simulink model "capsubot_Simulation_comparison_LandC"  (R2019a)
settings: Solver=ode45  StartTime=0.0  StopTime=16  FixedStep=.0001  MaxStep=.001  MinStep=.000001  RelTol=1e-3  EnableMultiTasking=on
values from neighbouring files (symbols this model uses):
  a1 = -a_stoke    [capsubot_dataperfectLuGree.m]
  a_c_desired_backward = [-a_all1' -a_all2']    [capsubot_dataperfectLuGree.m]
  a_u_desired = [a_all2' a_all1' a_all1' a_all2']    [capsubot_dataperfectLuGree.m]
  a_u_desired_backward = [-a_all2' -a_all1' -a_all1' -a_all2']    [capsubot_dataperfectLuGree.m]
  f_sm = data(8)    [capsubot_dataperfectLuGree.m]
  f_sM = 0.49    [capsubot_dataperfectLuGree.m]
  fv_Cap = data(9)    [capsubot_dataperfectLuGree.m]
  fv_IM = data(9)    [capsubot_dataperfectLuGree.m]
  g = 9.8    [capsubot_dataperfectLuGree.m]
  j = 30    [capsubot_dataperfectLuGree.m]
  k1 = 300    [capsubot_dataperfectLuGree.m]
  k2 = 100    [capsubot_dataperfectLuGree.m]
  m = data(2)    [capsubot_dataperfectLuGree.m]
  M = data(1)    [capsubot_dataperfectLuGree.m]
  m1 = data(2)    [capsubot_dataperfectLuGree.m]
  mu = data(3)    [capsubot_dataperfectLuGree.m]
  mu_1 = data(4)    [capsubot_dataperfectLuGree.m]
  mu_m = data(4)    [capsubot_dataperfectLuGree.m]
  sig_cap0 = data(8)    [capsubot_dataperfectLuGree.m]
  sig_cap1 = data(11)    [capsubot_dataperfectLuGree.m]
  sig_IM0 = data(8)    [capsubot_dataperfectLuGree.m]
  sig_IM1 = data(9)    [capsubot_dataperfectLuGree.m]
  tc = zeros(n,2)    [capsubot_dataperfectLuGree.m]
  tu = zeros(n,4)    [capsubot_dataperfectLuGree.m]
  z_cap = data(7)    [capsubot_dataperfectLuGree.m]
  z_IM = data(9)    [capsubot_dataperfectLuGree.m]
undefined symbols (not defined in the file or in its folder): profile, time_sim_individual_cum
libraries: fuzblock x2
(part 2 of 3)

== matlab function capsubot_Simulation_comparison_LandC/ Trajectory Tracking Controller/Selection Algorithm/Embedded MATLAB Function for the selection of acceleration	 ==
  data: u input; a_md output; tu parameter; time_sim_individual_cum parameter; profile parameter; a_u_desired parameter; a_c_desired_backward parameter; tc parameter; a_u_desired_backward parameter
function a_md  = fcn(u, tu, time_sim_individual_cum,profile,a_u_desired, a_c_desired_backward, tc, a_u_desired_backward )
 
t_add1=0;

%% 11111111111111111%%%%%%%%%%%%%%       %%%%    %%%%

if u<=(t_add1 + tu(profile(1),1))
        a_md =a_u_desired(profile(1),1) ;
elseif (u>(t_add1 + tu(profile(1),1))) && (u<=(t_add1 + tu(profile(1),2))) 
        a_md =a_u_desired(profile(1),2) ;
elseif (u>(t_add1 + tu(profile(1),2))) && (u<=(t_add1 + tu(profile(1),3))) 
        a_md =a_u_desired(profile(1),3) ;
elseif (u>(t_add1 + tu(profile(1),3))) && (u<=(t_add1 + tu(profile(1),4)))
             a_md =a_u_desired(profile(1),4) ;

elseif (u>(t_add1 + tu(profile(1),4))) && (u<=(tu(profile(1),4) + tu(profile(1),1)))
             a_md =a_u_desired(profile(1),1) ;                  
elseif (u>(tu(profile(1),4) + tu(profile(1),1))) && (u<=(tu(profile(1),4) + tu(profile(1),2)))
             a_md =a_u_desired(profile(1),2) ;
elseif (u>(tu(profile(1),4) + tu(profile(1),2))) && (u<=(tu(profile(1),4) + tu(profile(1),3)))
             a_md =a_u_desired(profile(1),3) ;   
elseif (u>(tu(profile(1),4) + tu(profile(1),3))) && (u<=(tu(profile(1),4) + tu(profile(1),4)))
             a_md =a_u_desired(profile(1),4) ;      

elseif (u>( tu(profile(1),4) + tu(profile(1),4))) && (u<=(2*tu(profile(1),4) + tu(profile(1),1)))
             a_md =a_u_desired(profile(1),1) ;                  
elseif (u>(2*tu(profile(1),4) + tu(profile(1),1))) && (u<=(2*tu(profile(1),4) + tu(profile(1),2)))
             a_md =a_u_desired(profile(1),2) ;
elseif (u>(2*tu(profile(1),4) + tu(profile(1),2))) && (u<=(2*tu(profile(1),4) + tu(profile(1),3)))
             a_md =a_u_desired(profile(1),3) ;   
elseif (u>(2*tu(profile(1),4) + tu(profile(1),3))) && (u<=(2*tu(profile(1),4) + tu(profile(1),4)))
             a_md =a_u_desired(profile(1),4) ;   

elseif (u>( 3*tu(profile(1),4) )) && (u<=(3*tu(profile(1),4) + tu(profile(1),1)))
             a_md =a_u_desired(profile(1),1) ;                  
elseif (u>(3*tu(profile(1),4) + tu(profile(1),1))) && (u<=(3*tu(profile(1),4) + tu(profile(1),2)))
             a_md =a_u_desired(profile(1),2) ;
elseif (u>(3*tu(profile(1),4) + tu(profile(1),2))) && (u<=(3*tu(profile(1),4) + tu(profile(1),3)))
             a_md =a_u_desired(profile(1),3) ;   
elseif (u>(3*tu(profile(1),4) + tu(profile(1),3))) && (u<=(3*tu(profile(1),4) + tu(profile(1),4)))
             a_md =a_u_desired(profile(1),4) ;                       

elseif (u>( 4*tu(profile(1),4) )) && (u<=(4*tu(profile(1),4) + tu(profile(1),1)))
             a_md =a_u_desired(profile(1),1) ;                  
elseif (u>(4*tu(profile(1),4) + tu(profile(1),1))) && (u<=(4*tu(profile(1),4) + tu(profile(1),2)))
             a_md =a_u_desired(profile(1),2) ;
elseif (u>(4*tu(profile(1),4) + tu(profile(1),2))) && (u<=(4*tu(profile(1),4) + tu(profile(1),3)))
             a_md =a_u_desired(profile(1),3) ;   
elseif (u>(4*tu(profile(1),4) + tu(profile(1),3))) && (u<=(4*tu(profile(1),4) + tu(profile(1),4)))
             a_md =a_u_desired(profile(1),4) ;    

elseif (u>( 5*tu(profile(1),4) )) && (u<=(4*tu(profile(1),4) + tu(profile(1),1)))
             a_md =a_u_desired(profile(1),1) ;                  
elseif (u>(4*tu(profile(1),4) + tu(profile(1),1))) && (u<=(4*tu(profile(1),4) + tu(profile(1),2)))
             a_md =a_u_desired(profile(1),2) ;
elseif (u>(4*tu(profile(1),4) + tu(profile(1),2))) && (u<=(4*tu(profile(1),4) + tu(profile(1),3)))
             a_md =a_u_desired(profile(1),3) ;   
elseif (u>(4*tu(profile(1),4) + tu(profile(1),3))) && (u<=(4*tu(profile(1),4) + tu(profile(1),4)))
             a_md =a_u_desired(profile(1),4) ;   


             
%% 22222222222222222 %%%%%%%%%%%%%%       %%%%    %%%%



elseif (u>( time_sim_individual_cum (1) )) && (u<=( time_sim_individual_cum(1) + tu(profile(2),1)))
             a_md =a_u_desired(profile(2),1) ;                  
elseif (u>( time_sim_individual_cum (1) + tu(profile(2),1) )) && (u<=( time_sim_individual_cum(1) + tu(profile(2),2)))
             a_md =a_u_desired(profile(2),2) ;
elseif (u>( time_sim_individual_cum (1) + tu(profile(2),2) )) && (u<=( time_sim_individual_cum(1) + tu(profile(2),3)))
             a_md =a_u_desired(profile(2),3) ;   
elseif (u>( time_sim_individual_cum (1) + tu(profile(2),3) )) && (u<=( time_sim_individual_cum(1) + tu(profile(2),4)))
             a_md =a_u_desired(profile(2),4) ;  

elseif (u>( time_sim_individual_cum (1) + 1*tu(profile(2),4) )) && (u<=(time_sim_individual_cum(1) + 1*tu(profile(2),4) + tu(profile(2),1)))
             a_md =a_u_desired(profile(2),1) ;                  
elseif (u>( time_sim_individual_cum (1) + 1*tu(profile(2),4) + tu(profile(2),1) )) && (u<=( time_sim_individual_cum(1) + 1*tu(profile(2),4) + tu(profile(2),2)))
             a_md =a_u_desired(profile(2),2) ;
elseif (u>( time_sim_individual_cum (1)+ 1*tu(profile(2),4) + tu(profile(2),2) )) && (u<=( time_sim_individual_cum(1)+ 1*tu(profile(2),4) + tu(profile(2),3)))
             a_md =a_u_desired(profile(2),3) ;   
elseif (u>( time_sim_individual_cum (1)+ 1*tu(profile(2),4) + tu(profile(2),3) )) && (u<=( time_sim_individual_cum(1)+ 1*tu(profile(2),4) + tu(profile(2),4)))
             a_md =a_u_desired(profile(2),4) ;                       


elseif (u>( time_sim_individual_cum (1) + 2*tu(profile(2),4) )) && (u<=(time_sim_individual_cum(1) + 2*tu(profile(2),4) + tu(profile(2),1)))
             a_md =a_u_desired(profile(2),1) ;                  
elseif (u>( time_sim_individual_cum (1) + 2*tu(profile(2),4) + tu(profile(2),1) )) && (u<=( time_sim_individual_cum(1) + 2*tu(profile(2),4) + tu(profile(2),2)))
             a_md =a_u_desired(profile(2),2) ;
elseif (u>( time_sim_individual_cum (1)+ 2*tu(profile(2),4) + tu(profile(2),2) )) && (u<=( time_sim_individual_cum(1)+ 2*tu(profile(2),4) + tu(profile(2),3)))
             a_md =a_u_desired(profile(2),3) ;   
elseif (u>( time_sim_individual_cum (1)+ 2*tu(profile(2),4) + tu(profile(2),3) )) && (u<=( time_sim_individual_cum(1)+ 2*tu(profile(2),4) + tu(profile(2),4)))
             a_md =a_u_desired(profile(2),4) ;                       
             

elseif (u>( time_sim_individual_cum (1) + 3*tu(profile(2),4) )) && (u<=(time_sim_individual_cum(1) + 3*tu(profile(2),4) + tu(profile(2),1)))
             a_md =a_u_desired(profile(2),1) ;                  
elseif (u>( time_sim_individual_cum (1) + 3*tu(profile(2),4) + tu(profile(2),1) )) && (u<=( time_sim_individual_cum(1) + 3*tu(profile(2),4) + tu(profile(2),2)))
             a_md =a_u_desired(profile(2),2) ;
elseif (u>( time_sim_individual_cum (1)+ 3*tu(profile(2),4) + tu(profile(2),2) )) && (u<=( time_sim_individual_cum(1)+ 3*tu(profile(2),4) + tu(profile(2),3)))
             a_md =a_u_desired(profile(2),3) ;   
elseif (u>( time_sim_individual_cum (1)+ 3*tu(profile(2),4) + tu(profile(2),3) )) && (u<=( time_sim_individual_cum(1)+ 3*tu(profile(2),4) + tu(profile(2),4)))
             a_md =a_u_desired(profile(2),4) ;               
             
             
elseif (u>( time_sim_individual_cum (1) + 4*tu(profile(2),4) )) && (u<=(time_sim_individual_cum(1) + 4*tu(profile(2),4) + tu(profile(2),1)))
             a_md =a_u_desired(profile(2),1) ;                  
elseif (u>( time_sim_individual_cum (1) + 4*tu(profile(2),4) + tu(profile(2),1) )) && (u<=( time_sim_individual_cum(1) + 4*tu(profile(2),4) + tu(profile(2),2)))
             a_md =a_u_desired(profile(2),2) ;
elseif (u>( time_sim_individual_cum (1)+ 4*tu(profile(2),4) + tu(profile(2),2) )) && (u<=( time_sim_individual_cum(1)+ 4*tu(profile(2),4) + tu(profile(2),3)))
             a_md =a_u_desired(profile(2),3) ;   
elseif (u>( time_sim_individual_cum (1)+ 4*tu(profile(2),4) + tu(profile(2),3) )) && (u<=( time_sim_individual_cum(1)+ 4*tu(profile(2),4) + tu(profile(2),4)))
             a_md =a_u_desired(profile(2),4) ; 
             
             

%% 33333333333333333333 %%%%%%%%%%%%%%       %%%%    %%%%             

             

elseif (u>( time_sim_individual_cum (2) + 0*tu(profile(3),4) )) && (u<=(time_sim_individual_cum(2) + 0*tu(profile(3),4) + tu(profile(3),1)))
             a_md =a_u_desired(profile(3),1) ;                  
elseif (u>( time_sim_individual_cum (2) + 0*tu(profile(3),4) + tu(profile(3),1) )) && (u<=( time_sim_individual_cum(2) + 0*tu(profile(3),4) + tu(profile(3),2)))
             a_md =a_u_desired(profile(3),2) ;
elseif (u>( time_sim_individual_cum (2)+ 0*tu(profile(3),4) + tu(profile(3),2) )) && (u<=( time_sim_individual_cum(2)+ 0*tu(profile(3),4) + tu(profile(3),3)))
             a_md =a_u_desired(profile(3),3) ;   
elseif (u>( time_sim_individual_cum (2)+ 0*tu(profile(3),4) + tu(profile(3),3) )) && (u<=( time_sim_individual_cum(2)+ 0*tu(profile(3),4) + tu(profile(3),4)))
             a_md =a_u_desired(profile(3),4) ;    
             
             
elseif (u>( time_sim_individual_cum (2) + 1*tu(profile(3),4) )) && (u<=(time_sim_individual_cum(2) + 1*tu(profile(3),4) + tu(profile(3),1)))
             a_md =a_u_desired(profile(3),1) ;                  
elseif (u>( time_sim_individual_cum (2) + 1*tu(profile(3),4) + tu(profile(3),1) )) && (u<=( time_sim_individual_cum(2) + 1*tu(profile(3),4) + tu(profile(3),2)))
             a_md =a_u_desired(profile(3),2) ;
elseif (u>( time_sim_individual_cum (2)+ 1*tu(profile(3),4) + tu(profile(3),2) )) && (u<=( time_sim_individual_cum(2)+ 1*tu(profile(3),4) + tu(profile(3),3)))
             a_md =a_u_desired(profile(3),3) ;   
elseif (u>( time_sim_individual_cum (2)+ 1*tu(profile(3),4) + tu(profile(3),3) )) && (u<=( time_sim_individual_cum(2)+ 1*tu(profile(3),4) + tu(profile(3),4)))
             a_md =a_u_desired(profile(3),4) ;     
             
             
elseif (u>( time_sim_individual_cum (2) + 2*tu(profile(3),4) )) && (u<=(time_sim_individual_cum(2) + 2*tu(profile(3),4) + tu(profile(3),1)))
             a_md =a_u_desired(profile(3),1) ;                  
elseif (u>( time_sim_individual_cum (2) + 2*tu(profile(3),4) + tu(profile(3),1) )) && (u<=( time_sim_individual_cum(2) + 2*tu(profile(3),4) + tu(profile(3),2)))
             a_md =a_u_desired(profile(3),2) ;
elseif (u>( time_sim_individual_cum (2)+ 2*tu(profile(3),4) + tu(profile(3),2) )) && (u<=( time_sim_individual_cum(2)+ 2*tu(profile(3),4) + tu(profile(3),3)))
             a_md =a_u_desired(profile(3),3) ;   
elseif (u>( time_sim_individual_cum (2)+ 2*tu(profile(3),4) + tu(profile(3),3) )) && (u<=( time_sim_individual_cum(2)+ 2*tu(profile(3),4) + tu(profile(3),4)))
             a_md =a_u_desired(profile(3),4) ;                
             
             
elseif (u>( time_sim_individual_cum (2) + 3*tu(profile(3),4) )) && (u<=(time_sim_individual_cum(2) + 3*tu(profile(3),4) + tu(profile(3),1)))
             a_md =a_u_desired(profile(3),1) ;                  
elseif (u>( time_sim_individual_cum (2) + 3*tu(profile(3),4) + tu(profile(3),1) )) && (u<=( time_sim_individual_cum(2) + 3*tu(profile(3),4) + tu(profile(3),2)))
             a_md =a_u_desired(profile(3),2) ;
elseif (u>( time_sim_individual_cum (2)+ 3*tu(profile(3),4) + tu(profile(3),2) )) && (u<=( time_sim_individual_cum(2)+ 3*tu(profile(3),4) + tu(profile(3),3)))
             a_md =a_u_desired(profile(3),3) ;   
elseif (u>( time_sim_individual_cum (2)+ 3*tu(profile(3),4) + tu(profile(3),3) )) && (u<=( time_sim_individual_cum(2)+ 3*tu(profile(3),4) + tu(profile(3),4)))
             a_md =a_u_desired(profile(3),4) ;   
             
             
elseif (u>( time_sim_individual_cum (2) + 4*tu(profile(3),4) )) && (u<=(time_sim_individual_cum(2) + 4*tu(profile(3),4) + tu(profile(3),1)))
             a_md =a_u_desired(profile(3),1) ;                  
elseif (u>( time_sim_individual_cum (2) + 4*tu(profile(3),4) + tu(profile(3),1) )) && (u<=( time_sim_individual_cum(2) + 4*tu(profile(3),4) + tu(profile(3),2)))
             a_md =a_u_desired(profile(3),2) ;
elseif (u>( time_sim_individual_cum (2)+ 4*tu(profile(3),4) + tu(profile(3),2) )) && (u<=( time_sim_individual_cum(2)+ 4*tu(profile(3),4) + tu(profile(3),3)))
             a_md =a_u_desired(profile(3),3) ;   
elseif (u>( time_sim_individual_cum (2)+ 4*tu(profile(3),4) + tu(profile(3),3) )) && (u<=( time_sim_individual_cum(2)+ 4*tu(profile(3),4) + tu(profile(3),4)))
             a_md =a_u_desired(profile(3),4) ;  
             
             
             
             
%% 44444444444444444444 %%%%%%%%%%%%%%       %%%%    %%%%               
             
             
             
             
elseif (u>( time_sim_individual_cum (3) + 0*tu(profile(4),4) )) && (u<=(time_sim_individual_cum(3) + 0*tu(profile(4),4) + tu(profile(4),1)))
             a_md =a_u_desired(profile(4),1) ;                  
elseif (u>( time_sim_individual_cum (3) + 0*tu(profile(4),4) + tu(profile(4),1) )) && (u<=( time_sim_individual_cum(3) + 0*tu(profile(4),4) + tu(profile(4),2)))
             a_md =a_u_desired(profile(4),2) ;
elseif (u>( time_sim_individual_cum (3)+ 0*tu(profile(4),4) + tu(profile(4),2) )) && (u<=( time_sim_individual_cum(3)+ 0*tu(profile(4),4) + tu(profile(4),3)))
             a_md =a_u_desired(profile(4),3) ;   
elseif (u>( time_sim_individual_cum (3)+ 0*tu(profile(4),4) + tu(profile(4),3) )) && (u<=( time_sim_individual_cum(3)+ 0*tu(profile(4),4) + tu(profile(4),4)))
             a_md =a_u_desired(profile(4),4) ;               
             
             
elseif (u>( time_sim_individual_cum (3) + 1*tu(profile(4),4) )) && (u<=(time_sim_individual_cum(3) + 1*tu(profile(4),4) + tu(profile(4),1)))
             a_md =a_u_desired(profile(4),1) ;                  
elseif (u>( time_sim_individual_cum (3) + 1*tu(profile(4),4) + tu(profile(4),1) )) && (u<=( time_sim_individual_cum(3) + 1*tu(profile(4),4) + tu(profile(4),2)))
             a_md =a_u_desired(profile(4),2) ;
elseif (u>( time_sim_individual_cum (3)+ 1*tu(profile(4),4) + tu(profile(4),2) )) && (u<=( time_sim_individual_cum(3)+ 1*tu(profile(4),4) + tu(profile(4),3)))
             a_md =a_u_desired(profile(4),3) ;   
elseif (u>( time_sim_individual_cum (3)+ 1*tu(profile(4),4) + tu(profile(4),3) )) && (u<=( time_sim_individual_cum(3)+ 1*tu(profile(4),4) + tu(profile(4),4)))
             a_md =a_u_desired(profile(4),4) ;   
             

elseif (u>( time_sim_individual_cum (3) + 2*tu(profile(4),4) )) && (u<=(time_sim_individual_cum(3) + 2*tu(profile(4),4) + tu(profile(4),1)))
             a_md =a_u_desired(profile(4),1) ;                  
elseif (u>( time_sim_individual_cum (3) + 2*tu(profile(4),4) + tu(profile(4),1) )) && (u<=( time_sim_individual_cum(3) + 2*tu(profile(4),4) + tu(profile(4),2)))
             a_md =a_u_desired(profile(4),2) ;
elseif (u>( time_sim_individual_cum (3)+ 2*tu(profile(4),4) + tu(profile(4),2) )) && (u<=( time_sim_individual_cum(3)+ 2*tu(profile(4),4) + tu(profile(4),3)))
             a_md =a_u_desired(profile(4),3) ;   
elseif (u>( time_sim_individual_cum (3)+ 2*tu(profile(4),4) + tu(profile(4),3) )) && (u<=( time_sim_individual_cum(3)+ 2*tu(profile(4),4) + tu(profile(4),4)))
             a_md =a_u_desired(profile(4),4) ;                
    
             
elseif (u>( time_sim_individual_cum (3) + 3*tu(profile(4),4) )) && (u<=(time_sim_individual_cum(3) + 3*tu(profile(4),4) + tu(profile(4),1)))
             a_md =a_u_desired(profile(4),1) ;                  
elseif (u>( time_sim_individual_cum (3) + 3*tu(profile(4),4) + tu(profile(4),1) )) && (u<=( time_sim_individual_cum(3) + 3*tu(profile(4),4) + tu(profile(4),2)))
             a_md =a_u_desired(profile(4),2) ;
elseif (u>( time_sim_individual_cum (3)+ 3*tu(profile(4),4) + tu(profile(4),2) )) && (u<=( time_sim_individual_cum(3)+ 3*tu(profile(4),4) + tu(profile(4),3)))
             a_md =a_u_desired(profile(4),3) ;   
elseif (u>( time_sim_individual_cum (3)+ 3*tu(profile(4),4) + tu(profile(4),3) )) && (u<=( time_sim_individual_cum(3)+ 3*tu(profile(4),4) + tu(profile(4),4)))
             a_md =a_u_desired(profile(4),4) ;                
             
             
             
%% 5555555555555555555555 %%%%%%%%%%%%%%       %%%%    %%%%               
             
             

elseif (u>( time_sim_individual_cum (4) + 0*tu(profile(5),4) )) && (u<=(time_sim_individual_cum(4) + 0*tu(profile(5),4) + tu(profile(5),1)))
             a_md =a_u_desired(profile(5),1) ;                  
elseif (u>( time_sim_individual_cum (4) + 0*tu(profile(5),4) + tu(profile(5),1) )) && (u<=( time_sim_individual_cum(4) + 0*tu(profile(5),4) + tu(profile(5),2)))
             a_md =a_u_desired(profile(5),2) ;
elseif (u>( time_sim_individual_cum (4)+ 0*tu(profile(5),4) + tu(profile(5),2) )) && (u<=( time_sim_individual_cum(4)+ 0*tu(profile(5),4) + tu(profile(5),3)))
             a_md =a_u_desired(profile(5),3) ;   
elseif (u>( time_sim_individual_cum (4)+ 0*tu(profile(5),4) + tu(profile(5),3) )) && (u<=( time_sim_individual_cum(4)+ 0*tu(profile(5),4) + tu(profile(5),4)))
             a_md =a_u_desired(profile(5),4) ;                 
             

elseif (u>( time_sim_individual_cum (4) + 1*tu(profile(5),4) )) && (u<=(time_sim_individual_cum(4) + 1*tu(profile(5),4) + tu(profile(5),1)))
             a_md =a_u_desired(profile(5),1) ;                  
elseif (u>( time_sim_individual_cum (4) + 1*tu(profile(5),4) + tu(profile(5),1) )) && (u<=( time_sim_individual_cum(4) + 1*tu(profile(5),4) + tu(profile(5),2)))
             a_md =a_u_desired(profile(5),2) ;
elseif (u>( time_sim_individual_cum (4)+ 1*tu(profile(5),4) + tu(profile(5),2) )) && (u<=( time_sim_individual_cum(4)+ 1*tu(profile(5),4) + tu(profile(5),3)))
             a_md =a_u_desired(profile(5),3) ;   
elseif (u>( time_sim_individual_cum (4)+ 1*tu(profile(5),4) + tu(profile(5),3) )) && (u<=( time_sim_individual_cum(4)+ 1*tu(profile(5),4) + tu(profile(5),4)))
             a_md =a_u_desired(profile(5),4) ;    

             
elseif (u>( time_sim_individual_cum (4) + 2*tu(profile(5),4) )) && (u<=(time_sim_individual_cum(4) + 2*tu(profile(5),4) + tu(profile(5),1)))
             a_md =a_u_desired(profile(5),1) ;                  
elseif (u>( time_sim_individual_cum (4) + 2*tu(profile(5),4) + tu(profile(5),1) )) && (u<=( time_sim_individual_cum(4) + 2*tu(profile(5),4) + tu(profile(5),2)))
             a_md =a_u_desired(profile(5),2) ;
elseif (u>( time_sim_individual_cum (4)+ 2*tu(profile(5),4) + tu(profile(5),2) )) && (u<=( time_sim_individual_cum(4)+ 2*tu(profile(5),4) + tu(profile(5),3)))
             a_md =a_u_desired(profile(5),3) ;   
elseif (u>( time_sim_individual_cum (4)+ 2*tu(profile(5),4) + tu(profile(5),3) )) && (u<=( time_sim_individual_cum(4)+ 2*tu(profile(5),4) + tu(profile(5),4)))
             a_md =a_u_desired(profile(5),4) ;              

             
elseif (u>( time_sim_individual_cum (4) + 3*tu(profile(5),4) )) && (u<=(time_sim_individual_cum(4) + 3*tu(profile(5),4) + tu(profile(5),1)))
             a_md =a_u_desired(profile(5),1) ;                  
elseif (u>( time_sim_individual_cum (4) + 3*tu(profile(5),4) + tu(profile(5),1) )) && (u<=( time_sim_individual_cum(4) + 3*tu(profile(5),4) + tu(profile(5),2)))
             a_md =a_u_desired(profile(5),2) ;
elseif (u>( time_sim_individual_cum (4)+ 3*tu(profile(5),4) + tu(profile(5),2) )) && (u<=( time_sim_individual_cum(4)+ 3*tu(profile(5),4) + tu(profile(5),3)))
             a_md =a_u_desired(profile(5),3) ;   
elseif (u>( time_sim_individual_cum (4)+ 3*tu(profile(5),4) + tu(profile(5),3) )) && (u<=( time_sim_individual_cum(4)+ 3*tu(profile(5),4) + tu(profile(5),4)))
             a_md =a_u_desired(profile(5),4) ;     
             

elseif (u>( time_sim_individual_cum (4) + 4*tu(profile(5),4) )) && (u<=(time_sim_individual_cum(4) + 4*tu(profile(5),4) + tu(profile(5),1)))
             a_md =a_u_desired(profile(5),1) ;                  
elseif (u>( time_sim_individual_cum (4) + 4*tu(profile(5),4) + tu(profile(5),1) )) && (u<=( time_sim_individual_cum(4) + 4*tu(profile(5),4) + tu(profile(5),2)))
             a_md =a_u_desired(profile(5),2) ;
elseif (u>( time_sim_individual_cum (4)+ 4*tu(profile(5),4) + tu(profile(5),2) )) && (u<=( time_sim_individual_cum(4)+ 4*tu(profile(5),4) + tu(profile(5),3)))
             a_md =a_u_desired(profile(5),3) ;   
elseif (u>( time_sim_individual_cum (4)+ 4*tu(profile(5),4) + tu(profile(5),3) )) && (u<=( time_sim_individual_cum(4)+ 4*tu(profile(5),4) + tu(profile(5),4)))
             a_md =a_u_desired(profile(5),4) ;    
             

             
%% 66666666666666666666 %%%%%%%%%%%%%%       %%%%    %%%%              
             
             
elseif (u>( time_sim_individual_cum (5) + 0*tu(profile(6),4) )) && (u<=(time_sim_individual_cum(5) + 0*tu(profile(6),4) + tu(profile(6),1)))
             a_md =a_u_desired(profile(6),1) ;                  
elseif (u>( time_sim_individual_cum (5) + 0*tu(profile(6),4) + tu(profile(6),1) )) && (u<=( time_sim_individual_cum(5) + 0*tu(profile(6),4) + tu(profile(6),2)))
             a_md =a_u_desired(profile(6),2) ;
elseif (u>( time_sim_individual_cum (5)+ 0*tu(profile(6),4) + tu(profile(6),2) )) && (u<=( time_sim_individual_cum(5)+ 0*tu(profile(6),4) + tu(profile(6),3)))
             a_md =a_u_desired(profile(6),3) ;   
elseif (u>( time_sim_individual_cum (5)+ 0*tu(profile(6),4) + tu(profile(6),3) )) && (u<=( time_sim_individual_cum(5)+ 0*tu(profile(6),4) + tu(profile(6),4)))
             a_md =a_u_desired(profile(6),4) ;   
             

elseif (u>( time_sim_individual_cum (5) + 1*tu(profile(6),4) )) && (u<=(time_sim_individual_cum(5) + 1*tu(profile(6),4) + tu(profile(6),1)))
             a_md =a_u_desired(profile(6),1) ;                  
elseif (u>( time_sim_individual_cum (5) + 1*tu(profile(6),4) + tu(profile(6),1) )) && (u<=( time_sim_individual_cum(5) + 1*tu(profile(6),4) + tu(profile(6),2)))
             a_md =a_u_desired(profile(6),2) ;
elseif (u>( time_sim_individual_cum (5)+ 1*tu(profile(6),4) + tu(profile(6),2) )) && (u<=( time_sim_individual_cum(5)+ 1*tu(profile(6),4) + tu(profile(6),3)))
             a_md =a_u_desired(profile(6),3) ;   
elseif (u>( time_sim_individual_cum (5)+ 1*tu(profile(6),4) + tu(profile(6),3) )) && (u<=( time_sim_individual_cum(5)+ 1*tu(profile(6),4) + tu(profile(6),4)))
             a_md =a_u_desired(profile(6),4) ;    
             
             
elseif (u>( time_sim_individual_cum (5) + 2*tu(profile(6),4) )) && (u<=(time_sim_individual_cum(5) + 2*tu(profile(6),4) + tu(profile(6),1)))
             a_md =a_u_desired(profile(6),1) ;                  
elseif (u>( time_sim_individual_cum (5) + 2*tu(profile(6),4) + tu(profile(6),1) )) && (u<=( time_sim_individual_cum(5) + 2*tu(profile(6),4) + tu(profile(6),2)))
             a_md =a_u_desired(profile(6),2) ;
elseif (u>( time_sim_individual_cum (5)+ 2*tu(profile(6),4) + tu(profile(6),2) )) && (u<=( time_sim_individual_cum(5)+ 2*tu(profile(6),4) + tu(profile(6),3)))
             a_md =a_u_desired(profile(6),3) ;   
elseif (u>( time_sim_individual_cum (5)+ 2*tu(profile(6),4) + tu(profile(6),3) )) && (u<=( time_sim_individual_cum(5)+ 2*tu(profile(6),4) + tu(profile(6),4)))
             a_md =a_u_desired(profile(6),4) ; 
             
             
elseif (u>( time_sim_individual_cum (5) + 3*tu(profile(6),4) )) && (u<=(time_sim_individual_cum(5) + 3*tu(profile(6),4) + tu(profile(6),1)))
             a_md =a_u_desired(profile(6),1) ;                  
elseif (u>( time_sim_individual_cum (5) + 3*tu(profile(6),4) + tu(profile(6),1) )) && (u<=( time_sim_individual_cum(5) + 3*tu(profile(6),4) + tu(profile(6),2)))
             a_md =a_u_desired(profile(6),2) ;
elseif (u>( time_sim_individual_cum (5)+ 3*tu(profile(6),4) + tu(profile(6),2) )) && (u<=( time_sim_individual_cum(5)+ 3*tu(profile(6),4) + tu(profile(6),3)))
             a_md =a_u_desired(profile(6),3) ;   
elseif (u>( time_sim_individual_cum (5)+ 3*tu(profile(6),4) + tu(profile(6),3) )) && (u<=( time_sim_individual_cum(5)+ 3*tu(profile(6),4) + tu(profile(6),4)))
             a_md =a_u_desired(profile(6),4) ;  
             
             
elseif (u>( time_sim_individual_cum (5) + 4*tu(profile(6),4) )) && (u<=(time_sim_individual_cum(5) + 4*tu(profile(6),4) + tu(profile(6),1)))
             a_md =a_u_desired(profile(6),1) ;                  
elseif (u>( time_sim_individual_cum (5) + 4*tu(profile(6),4) + tu(profile(6),1) )) && (u<=( time_sim_individual_cum(5) + 4*tu(profile(6),4) + tu(profile(6),2)))
             a_md =a_u_desired(profile(6),2) ;
elseif (u>( time_sim_individual_cum (5)+ 4*tu(profile(6),4) + tu(profile(6),2) )) && (u<=( time_sim_individual_cum(5)+ 4*tu(profile(6),4) + tu(profile(6),3)))
             a_md =a_u_desired(profile(6),3) ;   
elseif (u>( time_sim_individual_cum (5)+ 4*tu(profile(6),4) + tu(profile(6),3) )) && (u<=( time_sim_individual_cum(5)+ 4*tu(profile(6),4) + tu(profile(6),4)))
             a_md =a_u_desired(profile(6),4) ;              
             
             
             
%% 777777777777777 %%%%%%%%%%%%%%       %%%%    %%%%              
             
             
elseif (u>( time_sim_individual_cum (6) + 0*tu(profile(7),4) )) && (u<=(time_sim_individual_cum(6) + 0*tu(profile(7),4) + tu(profile(7),1)))
             a_md =a_u_desired(profile(7),1) ;                  
elseif (u>( time_sim_individual_cum (6) + 0*tu(profile(7),4) + tu(profile(7),1) )) && (u<=( time_sim_individual_cum(6) + 0*tu(profile(7),4) + tu(profile(7),2)))
             a_md =a_u_desired(profile(7),2) ;
elseif (u>( time_sim_individual_cum (6)+ 0*tu(profile(7),4) + tu(profile(7),2) )) && (u<=( time_sim_individual_cum(6)+ 0*tu(profile(7),4) + tu(profile(7),3)))
             a_md =a_u_desired(profile(7),3) ;   
elseif (u>( time_sim_individual_cum (6)+ 0*tu(profile(7),4) + tu(profile(7),3) )) && (u<=( time_sim_individual_cum(6)+ 0*tu(profile(7),4) + tu(profile(7),4)))
             a_md =a_u_desired(profile(7),4) ; 

elseif (u>( time_sim_individual_cum (6) + 1*tu(profile(7),4) )) && (u<=(time_sim_individual_cum(6) + 1*tu(profile(7),4) + tu(profile(7),1)))
             a_md =a_u_desired(profile(7),1) ;                  
elseif (u>( time_sim_individual_cum (6) + 1*tu(profile(7),4) + tu(profile(7),1) )) && (u<=( time_sim_individual_cum(6) + 1*tu(profile(7),4) + tu(profile(7),2)))
             a_md =a_u_desired(profile(7),2) ;
elseif (u>( time_sim_individual_cum (6)+ 1*tu(profile(7),4) + tu(profile(7),2) )) && (u<=( time_sim_individual_cum(6)+ 1*tu(profile(7),4) + tu(profile(7),3)))
             a_md =a_u_desired(profile(7),3) ;   
elseif (u>( time_sim_individual_cum (6)+ 1*tu(profile(7),4) + tu(profile(7),3) )) && (u<=( time_sim_individual_cum(6)+ 1*tu(profile(7),4) + tu(profile(7),4)))
             a_md =a_u_desired(profile(7),4) ; 
             
elseif (u>( time_sim_individual_cum (6) + 2*tu(profile(7),4) )) && (u<=(time_sim_individual_cum(6) + 2*tu(profile(7),4) + tu(profile(7),1)))
             a_md =a_u_desired(profile(7),1) ;                  
elseif (u>( time_sim_individual_cum (6) + 2*tu(profile(7),4) + tu(profile(7),1) )) && (u<=( time_sim_individual_cum(6) + 2*tu(profile(7),4) + tu(profile(7),2)))
             a_md =a_u_desired(profile(7),2) ;
elseif (u>( time_sim_individual_cum (6)+ 2*tu(profile(7),4) + tu(profile(7),2) )) && (u<=( time_sim_individual_cum(6)+ 2*tu(profile(7),4) + tu(profile(7),3)))
             a_md =a_u_desired(profile(7),3) ;   
elseif (u>( time_sim_individual_cum (6)+ 2*tu(profile(7),4) + tu(profile(7),3) )) && (u<=( time_sim_individual_cum(6)+ 2*tu(profile(7),4) + tu(profile(7),4)))
             a_md =a_u_desired(profile(7),4) ;      

             
elseif (u>( time_sim_individual_cum (6) + 3*tu(profile(7),4) )) && (u<=(time_sim_individual_cum(6) + 3*tu(profile(7),4) + tu(profile(7),1)))
             a_md =a_u_desired(profile(7),1) ;                  
elseif (u>( time_sim_individual_cum (6) + 3*tu(profile(7),4) + tu(profile(7),1) )) && (u<=( time_sim_individual_cum(6) + 3*tu(profile(7),4) + tu(profile(7),2)))
             a_md =a_u_desired(profile(7),2) ;
elseif (u>( time_sim_individual_cum (6)+ 3*tu(profile(7),4) + tu(profile(7),2) )) && (u<=( time_sim_individual_cum(6)+ 3*tu(profile(7),4) + tu(profile(7),3)))
             a_md =a_u_desired(profile(7),3) ;   
elseif (u>( time_sim_individual_cum (6)+ 3*tu(profile(7),4) + tu(profile(7),3) )) && (u<=( time_sim_individual_cum(6)+ 3*tu(profile(7),4) + tu(profile(7),4)))
             a_md =a_u_desired(profile(7),4) ;             
             
             

%% 88888888888888888888 %%%%%%%%%%%%%%       %%%%    %%%%              
                          
elseif (u>(time_sim_individual_cum (7) + 0*tu(profile(8),4) )) && (u<=(time_sim_individual_cum(7) + 0*tu(profile(7),4) + tu(profile(8),1)))
             a_md =a_u_desired(profile(8),1) ;                  
elseif (u>( time_sim_individual_cum (7) + 0*tu(profile(8),4) + tu(profile(8),1) )) && (u<=( time_sim_individual_cum(7) + 0*tu(profile(8),4) + tu(profile(8),2)))
             a_md =a_u_desired(profile(8),2) ;
elseif (u>( time_sim_individual_cum (7)+ 0*tu(profile(8),4) + tu(profile(8),2) )) && (u<=( time_sim_individual_cum(7)+ 0*tu(profile(8),4) + tu(profile(8),3)))
             a_md =a_u_desired(profile(8),3) ;   
elseif (u>( time_sim_individual_cum (7)+ 0*tu(profile(8),4) + tu(profile(8),3) )) && (u<=( time_sim_individual_cum(7)+ 0*tu(profile(8),4) + tu(profile(8),4)))
             a_md =a_u_desired(profile(8),4) ; 
             
elseif (u>(time_sim_individual_cum (7) + 1*tu(profile(8),4) )) && (u<=(time_sim_individual_cum(7) + 1*tu(profile(7),4) + tu(profile(8),1)))
             a_md =a_u_desired(profile(8),1) ;                  
elseif (u>( time_sim_individual_cum (7) + 1*tu(profile(8),4) + tu(profile(8),1) )) && (u<=( time_sim_individual_cum(7) + 1*tu(profile(8),4) + tu(profile(8),2)))
             a_md =a_u_desired(profile(8),2) ;
elseif (u>( time_sim_individual_cum (7)+ 1*tu(profile(8),4) + tu(profile(8),2) )) && (u<=( time_sim_individual_cum(7)+ 1*tu(profile(8),4) + tu(profile(8),3)))
             a_md =a_u_desired(profile(8),3) ;   
elseif (u>( time_sim_individual_cum (7)+ 1*tu(profile(8),4) + tu(profile(8),3) )) && (u<=( time_sim_individual_cum(7)+ 1*tu(profile(8),4) + tu(profile(8),4)))
             a_md =a_u_desired(profile(8),4) ;             
                          
elseif (u>(time_sim_individual_cum (7) + 2*tu(profile(8),4) )) && (u<=(time_sim_individual_cum(7) + 2*tu(profile(7),4) + tu(profile(8),1)))
             a_md =a_u_desired(profile(8),1) ;                  
elseif (u>( time_sim_individual_cum (7) + 2*tu(profile(8),4) + tu(profile(8),1) )) && (u<=( time_sim_individual_cum(7) + 2*tu(profile(8),4) + tu(profile(8),2)))
             a_md =a_u_desired(profile(8),2) ;
elseif (u>( time_sim_individual_cum (7)+ 2*tu(profile(8),4) + tu(profile(8),2) )) && (u<=( time_sim_individual_cum(7)+ 2*tu(profile(8),4) + tu(profile(8),3)))
             a_md =a_u_desired(profile(8),3) ;   
elseif (u>( time_sim_individual_cum (7)+ 2*tu(profile(8),4) + tu(profile(8),3) )) && (u<=( time_sim_individual_cum(7)+ 2*tu(profile(8),4) + tu(profile(8),4)))
             a_md =a_u_desired(profile(8),4) ;    
             
elseif (u>(time_sim_individual_cum (7) + 3*tu(profile(8),4) )) && (u<=(time_sim_individual_cum(7) + 3*tu(profile(7),4) + tu(profile(8),1)))
             a_md =a_u_desired(profile(8),1) ;                  
elseif (u>( time_sim_individual_cum (7) + 3*tu(profile(8),4) + tu(profile(8),1) )) && (u<=( time_sim_individual_cum(7) + 3*tu(profile(8),4) + tu(profile(8),2)))
             a_md =a_u_desired(profile(8),2) ;
elseif (u>( time_sim_individual_cum (7)+ 3*tu(profile(8),4) + tu(profile(8),2) )) && (u<=( time_sim_individual_cum(7)+ 3*tu(profile(8),4) + tu(profile(8),3)))
             a_md =a_u_desired(profile(8),3) ;   
elseif (u>( time_sim_individual_cum (7)+ 3*tu(profile(8),4) + tu(profile(8),3) )) && (u<=( time_sim_individual_cum(7)+ 3*tu(profile(8),4) + tu(profile(8),4)))
             a_md =a_u_desired(profile(8),4) ;  
             
elseif (u>(time_sim_individual_cum (7) + 4*tu(profile(8),4) )) && (u<=(time_sim_individual_cum(7) + 4*tu(profile(7),4) + tu(profile(8),1)))
             a_md =a_u_desired(profile(8),1) ;                  
elseif (u>( time_sim_individual_cum (7) + 4*tu(profile(8),4) + tu(profile(8),1) )) && (u<=( time_sim_individual_cum(7) + 4*tu(profile(8),4) + tu(profile(8),2)))
             a_md =a_u_desired(profile(8),2) ;
elseif (u>( time_sim_individual_cum (7)+ 4*tu(profile(8),4) + tu(profile(8),2) )) && (u<=( time_sim_individual_cum(7)+ 4*tu(profile(8),4) + tu(profile(8),3)))
             a_md =a_u_desired(profile(8),3) ;   
elseif (u>( time_sim_individual_cum (7)+ 4*tu(profile(8),4) + tu(profile(8),3) )) && (u<=( time_sim_individual_cum(7)+ 4*tu(profile(8),4) + tu(profile(8),4)))
             a_md =a_u_desired(profile(8),4) ;    
             
             
             
%%%%%%%%%%%%%%%%%%%%%%%%%%%%%%%%%%%%%%%%%%%%%%%%%%%%%%%%%%%%%%%%%%       
             
%% 9999999999999999999  %%%%%%%%%%%%%%       %%%%    %%%%          
             
elseif (u>(time_sim_individual_cum (8) + 0*tu(profile(8),4) )) && (u<=(time_sim_individual_cum(8) + 0*tu(profile(7),4) + tc(profile(9),1)))
             a_md =a_c_desired_backward(profile(9),1) ;                  
elseif (u>( time_sim_individual_cum (8) + 0*tu(profile(8),4) + tc(profile(8),1) )) && (u<=( time_sim_individual_cum(8) + 0*tu(profile(8),4) + tc(profile(9),2)))
             a_md =a_c_desired_backward(profile(9),2) ;

             
             
%%%%%%%%%%%%%%%%%%%%%%%%%%%%%%%%%%%%%%%%%%%%%%%%%%%%%%%%%%%%%%%%%%%      



%% 10 10 10 10 10 10  %%%%%%%%%%%%%%       %%%%    %%%% 

elseif (u>(time_sim_individual_cum (9) + 0*tu(profile(10),4) )) && (u<=(time_sim_individual_cum(9) + 0*tu(profile(10),4) + tu(profile(10),1)))
             a_md =a_u_desired_backward(profile(10),1) ;                  
elseif (u>( time_sim_individual_cum (9) + 0*tu(profile(10),4) + tu(profile(10),1) )) && (u<=( time_sim_individual_cum(9) + 0*tu(profile(10),4) + tu(profile(10),2)))
             a_md =a_u_desired_backward(profile(10),2) ;
elseif (u>( time_sim_individual_cum (9)+ 0*tu(profile(10),4) + tu(profile(10),2) )) && (u<=( time_sim_individual_cum(9)+ 0*tu(profile(10),4) + tu(profile(10),3)))
             a_md =a_u_desired_backward(profile(10),3) ;   
elseif (u>( time_sim_individual_cum (9)+ 0*tu(profile(10),4) + tu(profile(10),3) )) && (u<=( time_sim_individual_cum(9)+ 0*tu(profile(10),4) + tu(profile(10),4)))
             a_md =a_u_desired_backward(profile(10),4) ; 

elseif (u>(time_sim_individual_cum (9) + 1*tu(profile(10),4) )) && (u<=(time_sim_individual_cum(9) + 1*tu(profile(10),4) + tu(profile(10),1)))
             a_md =a_u_desired_backward(profile(10),1) ;                  
elseif (u>( time_sim_individual_cum (9) + 1*tu(profile(10),4) + tu(profile(10),1) )) && (u<=( time_sim_individual_cum(9) + 1*tu(profile(10),4) + tu(profile(10),2)))
             a_md =a_u_desired_backward(profile(10),2) ;
elseif (u>( time_sim_individual_cum (9)+ 1*tu(profile(10),4) + tu(profile(10),2) )) && (u<=( time_sim_individual_cum(9)+ 1*tu(profile(10),4) + tu(profile(10),3)))
             a_md =a_u_desired_backward(profile(10),3) ;   
elseif (u>( time_sim_individual_cum (9)+ 1*tu(profile(10),4) + tu(profile(10),3) )) && (u<=( time_sim_individual_cum(9)+ 1*tu(profile(10),4) + tu(profile(10),4)))
             a_md =a_u_desired_backward(profile(10),4) ; 
             
elseif (u>(time_sim_individual_cum (9) + 2*tu(profile(10),4) )) && (u<=(time_sim_individual_cum(9) + 2*tu(profile(10),4) + tu(profile(10),1)))
             a_md =a_u_desired_backward(profile(10),1) ;                  
elseif (u>( time_sim_individual_cum (9) + 2*tu(profile(10),4) + tu(profile(10),1) )) && (u<=( time_sim_individual_cum(9) + 2*tu(profile(10),4) + tu(profile(10),2)))
             a_md =a_u_desired_backward(profile(10),2) ;
elseif (u>( time_sim_individual_cum (9)+ 2*tu(profile(10),4) + tu(profile(10),2) )) && (u<=( time_sim_individual_cum(9)+ 2*tu(profile(10),4) + tu(profile(10),3)))
             a_md =a_u_desired_backward(profile(10),3) ;   
elseif (u>( time_sim_individual_cum (9)+ 2*tu(profile(10),4) + tu(profile(10),3) )) && (u<=( time_sim_individual_cum(9)+ 2*tu(profile(10),4) + tu(profile(10),4)))
             a_md =a_u_desired_backward(profile(10),4) ; 
             
elseif (u>(time_sim_individual_cum (9) + 3*tu(profile(10),4) )) && (u<=(time_sim_individual_cum(9) + 3*tu(profile(10),4) + tu(profile(10),1)))
             a_md =a_u_desired_backward(profile(10),1) ;                  
elseif (u>( time_sim_individual_cum (9) + 3*tu(profile(10),4) + tu(profile(10),1) )) && (u<=( time_sim_individual_cum(9) + 3*tu(profile(10),4) + tu(profile(10),2)))
             a_md =a_u_desired_backward(profile(10),2) ;
elseif (u>( time_sim_individual_cum (9)+ 3*tu(profile(10),4) + tu(profile(10),2) )) && (u<=( time_sim_individual_cum(9)+ 3*tu(profile(10),4) + tu(profile(10),3)))
             a_md =a_u_desired_backward(profile(10),3) ;   
elseif (u>( time_sim_individual_cum (9)+ 3*tu(profile(10),4) + tu(profile(10),3) )) && (u<=( time_sim_individual_cum(9)+ 3*tu(profile(10),4) + tu(profile(10),4)))
             a_md =a_u_desired_backward(profile(10),4) ;      
             
elseif (u>(time_sim_individual_cum (9) + 4*tu(profile(10),4) )) && (u<=(time_sim_individual_cum(9) + 4*tu(profile(10),4) + tu(profile(10),1)))
             a_md =a_u_desired_backward(profile(10),1) ;                  
elseif (u>( time_sim_individual_cum (9) + 4*tu(profile(10),4) + tu(profile(10),1) )) && (u<=( time_sim_individual_cum(9) + 4*tu(profile(10),4) + tu(profile(10),2)))
             a_md =a_u_desired_backward(profile(10),2) ;
elseif (u>( time_sim_individual_cum (9)+ 4*tu(profile(10),4) + tu(profile(10),2) )) && (u<=( time_sim_individual_cum(9)+ 4*tu(profile(10),4) + tu(profile(10),3)))
             a_md =a_u_desired_backward(profile(10),3) ;   
elseif (u>( time_sim_individual_cum (9)+ 4*tu(profile(10),4) + tu(profile(10),3) )) && (u<=( time_sim_individual_cum(9)+ 4*tu(profile(10),4) + tu(profile(10),4)))
             a_md =a_u_desired_backward(profile(10),4) ;              
             
elseif (u>(time_sim_individual_cum (9) + 5*tu(profile(10),4) )) && (u<=(time_sim_individual_cum(9) + 5*tu(profile(10),4) + tu(profile(10),1)))
             a_md =a_u_desired_backward(profile(10),1) ;                  
elseif (u>( time_sim_individual_cum (9) + 5*tu(profile(10),4) + tu(profile(10),1) )) && (u<=( time_sim_individual_cum(9) + 5*tu(profile(10),4) + tu(profile(10),2)))
             a_md =a_u_desired_backward(profile(10),2) ;
elseif (u>( time_sim_individual_cum (9)+ 5*tu(profile(10),4) + tu(profile(10),2) )) && (u<=( time_sim_individual_cum(9)+ 5*tu(profile(10),4) + tu(profile(10),3)))
             a_md =a_u_desired_backward(profile(10),3) ;   
elseif (u>( time_sim_individual_cum (9)+ 5*tu(profile(10),4) + tu(profile(10),3) )) && (u<=( time_sim_individual_cum(9)+ 5*tu(profile(10),4) + tu(profile(10),4)))
             a_md =a_u_desired_backward(profile(10),4) ;  
             
elseif (u>(time_sim_individual_cum (9) + 6*tu(profile(10),4) )) && (u<=(time_sim_individual_cum(9) + 6*tu(profile(10),4) + tu(profile(10),1)))
             a_md =a_u_desired_backward(profile(10),1) ;                  
elseif (u>( time_sim_individual_cum (9) + 6*tu(profile(10),4) + tu(profile(10),1) )) && (u<=( time_sim_individual_cum(9) + 6*tu(profile(10),4) + tu(profile(10),2)))
             a_md =a_u_desired_backward(profile(10),2) ;
elseif (u>( time_sim_individual_cum (9)+ 6*tu(profile(10),4) + tu(profile(10),2) )) && (u<=( time_sim_individual_cum(9)+ 6*tu(profile(10),4) + tu(profile(10),3)))
             a_md =a_u_desired_backward(profile(10),3) ;   
elseif (u>( time_sim_individual_cum (9)+ 6*tu(profile(10),4) + tu(profile(10),3) )) && (u<=( time_sim_individual_cum(9)+ 6*tu(profile(10),4) + tu(profile(10),4)))
             a_md =a_u_desired_backward(profile(10),4);  
             
elseif (u>(time_sim_individual_cum (9) + 7*tu(profile(10),4) )) && (u<=(time_sim_individual_cum(9) + 7*tu(profile(10),4) + tu(profile(10),1)))
             a_md =a_u_desired_backward(profile(10),1) ;                  
elseif (u>( time_sim_individual_cum (9) + 7*tu(profile(10),4) + tu(profile(10),1) )) && (u<=( time_sim_individual_cum(9) + 7*tu(profile(10),4) + tu(profile(10),2)))
             a_md =a_u_desired_backward(profile(10),2) ;
elseif (u>( time_sim_individual_cum (9)+ 7*tu(profile(10),4) + tu(profile(10),2) )) && (u<=( time_sim_individual_cum(9)+ 7*tu(profile(10),4) + tu(profile(10),3)))
             a_md =a_u_desired_backward(profile(10),3) ;   
elseif (u>( time_sim_individual_cum (9)+ 7*tu(profile(10),4) + tu(profile(10),3) )) && (u<=( time_sim_individual_cum(9)+ 7*tu(profile(10),4) + tu(profile(10),4)))
             a_md =a_u_desired_backward(profile(10),4) ;   
             
elseif (u>(time_sim_individual_cum (9) + 8*tu(profile(10),4) )) && (u<=(time_sim_individual_cum(9) + 8*tu(profile(10),4) + tu(profile(10),1)))
             a_md =a_u_desired_backward(profile(10),1) ;                  
elseif (u>( time_sim_individual_cum (9) + 8*tu(profile(10),4) + tu(profile(10),1) )) && (u<=( time_sim_individual_cum(9) + 8*tu(profile(10),4) + tu(profile(10),2)))
             a_md =a_u_desired_backward(profile(10),2) ;
elseif (u>( time_sim_individual_cum (9)+ 8*tu(profile(10),4) + tu(profile(10),2) )) && (u<=( time_sim_individual_cum(9)+ 8*tu(profile(10),4) + tu(profile(10),3)))
             a_md =a_u_desired_backward(profile(10),3) ;   
elseif (u>( time_sim_individual_cum (9)+ 8*tu(profile(10),4) + tu(profile(10),3) )) && (u<=( time_sim_individual_cum(9)+ 8*tu(profile(10),4) + tu(profile(10),4)))
             a_md =a_u_desired_backward(profile(10),4) ;    
             
                          
             
             
%% 11 11 11 11 11 11  %%%%%%%%%%%%%%       %%%%    %%%%              

elseif (u>(time_sim_individual_cum (10) + 0*tu(profile(11),4) )) && (u<=(time_sim_individual_cum(10) + 0*tu(profile(11),4) + tu(profile(11),1)))
             a_md =a_u_desired_backward(profile(11),1) ;                  
elseif (u>( time_sim_individual_cum (10) + 0*tu(profile(11),4) + tu(profile(11),1) )) && (u<=( time_sim_individual_cum(10) + 0*tu(profile(11),4) + tu(profile(11),2)))
             a_md =a_u_desired_backward(profile(11),2) ;
elseif (u>( time_sim_individual_cum (10)+ 0*tu(profile(11),4) + tu(profile(11),2) )) && (u<=( time_sim_individual_cum(10)+ 0*tu(profile(11),4) + tu(profile(11),3)))
             a_md =a_u_desired_backward(profile(11),3) ;   
elseif (u>( time_sim_individual_cum (10)+ 0*tu(profile(11),4) + tu(profile(11),3) )) && (u<=( time_sim_individual_cum(10)+ 0*tu(profile(11),4) + tu(profile(11),4)))
             a_md =a_u_desired_backward(profile(11),4) ;              
             
elseif (u>(time_sim_individual_cum (10) + 1*tu(profile(11),4) )) && (u<=(time_sim_individual_cum(10) + 1*tu(profile(11),4) + tu(profile(11),1)))
             a_md =a_u_desired_backward(profile(11),1) ;                  
elseif (u>( time_sim_individual_cum (10) + 1*tu(profile(11),4) + tu(profile(11),1) )) && (u<=( time_sim_individual_cum(10) + 1*tu(profile(11),4) + tu(profile(11),2)))
             a_md =a_u_desired_backward(profile(11),2) ;
elseif (u>( time_sim_individual_cum (10)+ 1*tu(profile(11),4) + tu(profile(11),2) )) && (u<=( time_sim_individual_cum(10)+ 1*tu(profile(11),4) + tu(profile(11),3)))
             a_md =a_u_desired_backward(profile(11),3) ;   
elseif (u>( time_sim_individual_cum (10)+ 1*tu(profile(11),4) + tu(profile(11),3) )) && (u<=( time_sim_individual_cum(10)+ 1*tu(profile(11),4) + tu(profile(11),4)))
             a_md =a_u_desired_backward(profile(11),4) ; 
             
elseif (u>(time_sim_individual_cum (10) + 2*tu(profile(11),4) )) && (u<=(time_sim_individual_cum(10) + 2*tu(profile(11),4) + tu(profile(11),1)))
             a_md =a_u_desired_backward(profile(11),1) ;                  
elseif (u>( time_sim_individual_cum (10) + 2*tu(profile(11),4) + tu(profile(11),1) )) && (u<=( time_sim_individual_cum(10) + 2*tu(profile(11),4) + tu(profile(11),2)))
             a_md =a_u_desired_backward(profile(11),2) ;
elseif (u>( time_sim_individual_cum (10)+ 2*tu(profile(11),4) + tu(profile(11),2) )) && (u<=( time_sim_individual_cum(10)+ 2*tu(profile(11),4) + tu(profile(11),3)))
             a_md =a_u_desired_backward(profile(11),3) ;   
elseif (u>( time_sim_individual_cum (10)+ 2*tu(profile(11),4) + tu(profile(11),3) )) && (u<=( time_sim_individual_cum(10)+ 2*tu(profile(11),4) + tu(profile(11),4)))
             a_md =a_u_desired_backward(profile(11),4) ;               
             
elseif (u>(time_sim_individual_cum (10) + 3*tu(profile(11),4) )) && (u<=(time_sim_individual_cum(10) + 3*tu(profile(11),4) + tu(profile(11),1)))
             a_md =a_u_desired_backward(profile(11),1) ;                  
elseif (u>( time_sim_individual_cum (10) + 3*tu(profile(11),4) + tu(profile(11),1) )) && (u<=( time_sim_individual_cum(10) + 3*tu(profile(11),4) + tu(profile(11),2)))
             a_md =a_u_desired_backward(profile(11),2) ;
elseif (u>( time_sim_individual_cum (10)+ 3*tu(profile(11),4) + tu(profile(11),2) )) && (u<=( time_sim_individual_cum(10)+ 3*tu(profile(11),4) + tu(profile(11),3)))
             a_md =a_u_desired_backward(profile(11),3) ;   
elseif (u>( time_sim_individual_cum (10)+ 3*tu(profile(11),4) + tu(profile(11),3) )) && (u<=( time_sim_individual_cum(10)+ 3*tu(profile(11),4) + tu(profile(11),4)))
             a_md =a_u_desired_backward(profile(11),4) ; 
             
             
%% 12 12 12 12 12 12  %%%%%%%%%%%%%%       %%%%    %%%%              
             
elseif (u>(time_sim_individual_cum (11) + 0*tu(profile(12),4) )) && (u<=(time_sim_individual_cum(11) + 0*tu(profile(12),4) + tu(profile(12),1)))
             a_md =a_u_desired_backward(profile(12),1) ;                  
elseif (u>( time_sim_individual_cum (11) + 0*tu(profile(12),4) + tu(profile(12),1) )) && (u<=( time_sim_individual_cum(11) + 0*tu(profile(12),4) + tu(profile(12),2)))
             a_md =a_u_desired_backward(profile(12),2) ;
elseif (u>( time_sim_individual_cum (11)+ 0*tu(profile(12),4) + tu(profile(12),2) )) && (u<=( time_sim_individual_cum(11)+ 0*tu(profile(12),4) + tu(profile(12),3)))
             a_md =a_u_desired_backward(profile(12),3) ;   
elseif (u>( time_sim_individual_cum (11)+ 0*tu(profile(12),4) + tu(profile(12),3) )) && (u<=( time_sim_individual_cum(11)+ 0*tu(profile(12),4) + tu(profile(12),4)))
             a_md =a_u_desired_backward(profile(12),4) ;               
             
elseif (u>(time_sim_individual_cum (11) + 1*tu(profile(12),4) )) && (u<=(time_sim_individual_cum(11) + 1*tu(profile(12),4) + tu(profile(12),1)))
             a_md =a_u_desired_backward(profile(12),1) ;                  
elseif (u>( time_sim_individual_cum (11) + 1*tu(profile(12),4) + tu(profile(12),1) )) && (u<=( time_sim_individual_cum(11) + 1*tu(profile(12),4) + tu(profile(12),2)))
             a_md =a_u_desired_backward(profile(12),2) ;
elseif (u>( time_sim_individual_cum (11)+ 1*tu(profile(12),4) + tu(profile(12),2) )) && (u<=( time_sim_individual_cum(11)+ 1*tu(profile(12),4) + tu(profile(12),3)))
             a_md =a_u_desired_backward(profile(12),3) ;   
elseif (u>( time_sim_individual_cum (11)+ 1*tu(profile(12),4) + tu(profile(12),3) )) && (u<=( time_sim_individual_cum(11)+ 1*tu(profile(12),4) + tu(profile(12),4)))
             a_md =a_u_desired_backward(profile(12),4) ;    
             
elseif (u>(time_sim_individual_cum (11) + 2*tu(profile(12),4) )) && (u<=(time_sim_individual_cum(11) + 2*tu(profile(12),4) + tu(profile(12),1)))
             a_md =a_u_desired_backward(profile(12),1) ;                  
elseif (u>( time_sim_individual_cum (11) + 2*tu(profile(12),4) + tu(profile(12),1) )) && (u<=( time_sim_individual_cum(11) + 2*tu(profile(12),4) + tu(profile(12),2)))
             a_md =a_u_desired_backward(profile(12),2) ;
elseif (u>( time_sim_individual_cum (11)+ 2*tu(profile(12),4) + tu(profile(12),2) )) && (u<=( time_sim_individual_cum(11)+ 2*tu(profile(12),4) + tu(profile(12),3)))
             a_md =a_u_desired_backward(profile(12),3) ;   
elseif (u>( time_sim_individual_cum (11)+ 2*tu(profile(12),4) + tu(profile(12),3) )) && (u<=( time_sim_individual_cum(11)+ 2*tu(profile(12),4) + tu(profile(12),4)))
             a_md =a_u_desired_backward(profile(12),4) ;  
             
elseif (u>(time_sim_individual_cum (11) + 3*tu(profile(12),4) )) && (u<=(time_sim_individual_cum(11) + 3*tu(profile(12),4) + tu(profile(12),1)))
             a_md =a_u_desired_backward(profile(12),1) ;                  
elseif (u>( time_sim_individual_cum (11) + 3*tu(profile(12),4) + tu(profile(12),1) )) && (u<=( time_sim_individual_cum(11) + 3*tu(profile(12),4) + tu(profile(12),2)))
             a_md =a_u_desired_backward(profile(12),2) ;
elseif (u>( time_sim_individual_cum (11)+ 3*tu(profile(12),4) + tu(profile(12),2) )) && (u<=( time_sim_individual_cum(11)+ 3*tu(profile(12),4) + tu(profile(12),3)))
             a_md =a_u_desired_backward(profile(12),3) ;   
elseif (u>( time_sim_individual_cum (11)+ 3*tu(profile(12),4) + tu(profile(12),3) )) && (u<=( time_sim_individual_cum(11)+ 3*tu(profile(12),4) + tu(profile(12),4)))
             a_md =a_u_desired_backward(profile(12),4) ;                
            
elseif (u>(time_sim_individual_cum (11) + 4*tu(profile(12),4) )) && (u<=(time_sim_individual_cum(11) + 4*tu(profile(12),4) + tu(profile(12),1)))
             a_md =a_u_desired_backward(profile(12),1) ;                  
elseif (u>( time_sim_individual_cum (11) + 4*tu(profile(12),4) + tu(profile(12),1) )) && (u<=( time_sim_individual_cum(11) + 4*tu(profile(12),4) + tu(profile(12),2)))
             a_md =a_u_desired_backward(profile(12),2) ;
elseif (u>( time_sim_individual_cum (11)+ 4*tu(profile(12),4) + tu(profile(12),2) )) && (u<=( time_sim_individual_cum(11)+ 4*tu(profile(12),4) + tu(profile(12),3)))
             a_md =a_u_desired_backward(profile(12),3) ;   
elseif (u>( time_sim_individual_cum (11)+ 4*tu(profile(12),4) + tu(profile(12),3) )) && (u<=( time_sim_individual_cum(11)+ 4*tu(profile(12),4) + tu(profile(12),4)))
             a_md =a_u_desired_backward(profile(12),4) ;   
             
             

%% 13 13 13 13 13 13  %%%%%%%%%%%%%%       %%%%    %%%%              
             
             
elseif (u>(time_sim_individual_cum (12) + 0*tu(profile(13),4) + 0*tu(profile(12),1))) && (u<=(time_sim_individual_cum(12) + 0*tu(profile(13),4) + tu(profile(13),1)))
             a_md =a_u_desired_backward(profile(13),1) ;                  
elseif (u>( time_sim_individual_cum (12) + 0*tu(profile(13),4) + tu(profile(13),1) )) && (u<=( time_sim_individual_cum(12) + 0*tu(profile(13),4) + tu(profile(13),2)))
             a_md =a_u_desired_backward(profile(13),2) ;
elseif (u>( time_sim_individual_cum (12)+ 0*tu(profile(13),4) + tu(profile(13),2) )) && (u<=( time_sim_individual_cum(12)+ 0*tu(profile(13),4) + tu(profile(13),3)))
             a_md =a_u_desired_backward(profile(13),3) ;   
elseif (u>( time_sim_individual_cum (12)+ 0*tu(profile(13),4) + tu(profile(13),3) )) && (u<=( time_sim_individual_cum(12)+ 0*tu(profile(13),4) + tu(profile(13),4)))
             a_md =a_u_desired_backward(profile(13),4) ;    
             
elseif (u>(time_sim_individual_cum (12) + 1*tu(profile(13),4) + 0*tu(profile(12),1))) && (u<=(time_sim_individual_cum(12) + 1*tu(profile(13),4) + tu(profile(13),1)))
             a_md =a_u_desired_backward(profile(13),1) ;                  
elseif (u>( time_sim_individual_cum (12) + 1*tu(profile(13),4) + tu(profile(13),1) )) && (u<=( time_sim_individual_cum(12) + 1*tu(profile(13),4) + tu(profile(13),2)))
             a_md =a_u_desired_backward(profile(13),2) ;
elseif (u>( time_sim_individual_cum (12)+ 1*tu(profile(13),4) + tu(profile(13),2) )) && (u<=( time_sim_individual_cum(12)+ 1*tu(profile(13),4) + tu(profile(13),3)))
             a_md =a_u_desired_backward(profile(13),3) ;   
elseif (u>( time_sim_individual_cum (12)+ 1*tu(profile(13),4) + tu(profile(13),3) )) && (u<=( time_sim_individual_cum(12)+ 1*tu(profile(13),4) + tu(profile(13),4)))
             a_md =a_u_desired_backward(profile(13),4) ;             
             
elseif (u>(time_sim_individual_cum (12) + 2*tu(profile(13),4) + 0*tu(profile(12),1))) && (u<=(time_sim_individual_cum(12) + 2*tu(profile(13),4) + tu(profile(13),1)))
             a_md =a_u_desired_backward(profile(13),1) ;                  
elseif (u>( time_sim_individual_cum (12) + 2*tu(profile(13),4) + tu(profile(13),1) )) && (u<=( time_sim_individual_cum(12) + 2*tu(profile(13),4) + tu(profile(13),2)))
             a_md =a_u_desired_backward(profile(13),2) ;
elseif (u>( time_sim_individual_cum (12)+ 2*tu(profile(13),4) + tu(profile(13),2) )) && (u<=( time_sim_individual_cum(12)+ 2*tu(profile(13),4) + tu(profile(13),3)))
             a_md =a_u_desired_backward(profile(13),3) ;   
elseif (u>( time_sim_individual_cum (12)+ 2*tu(profile(13),4) + tu(profile(13),3) )) && (u<=( time_sim_individual_cum(12)+ 2*tu(profile(13),4) + tu(profile(13),4)))
             a_md =a_u_desired_backward(profile(13),4) ;    
             
elseif (u>(time_sim_individual_cum (12) + 3*tu(profile(13),4) + 0*tu(profile(12),1))) && (u<=(time_sim_individual_cum(12) + 3*tu(profile(13),4) + tu(profile(13),1)))
             a_md =a_u_desired_backward(profile(13),1) ;                  
elseif (u>( time_sim_individual_cum (12) + 3*tu(profile(13),4) + tu(profile(13),1) )) && (u<=( time_sim_individual_cum(12) + 3*tu(profile(13),4) + tu(profile(13),2)))
             a_md =a_u_desired_backward(profile(13),2) ;
elseif (u>( time_sim_individual_cum (12)+ 3*tu(profile(13),4) + tu(profile(13),2) )) && (u<=( time_sim_individual_cum(12)+ 3*tu(profile(13),4) + tu(profile(13),3)))
             a_md =a_u_desired_backward(profile(13),3) ;   
elseif (u>( time_sim_individual_cum (12)+ 3*tu(profile(13),4) + tu(profile(13),3) )) && (u<=( time_sim_individual_cum(12)+ 3*tu(profile(13),4) + tu(profile(13),4)))
             a_md =a_u_desired_backward(profile(13),4) ;  
             
elseif (u>(time_sim_individual_cum (12) + 4*tu(profile(13),4) + 0*tu(profile(12),1))) && (u<=(time_sim_individual_cum(12) + 4*tu(profile(13),4) + tu(profile(13),1)))
             a_md =a_u_desired_backward(profile(13),1) ;                  
elseif (u>( time_sim_individual_cum (12) + 4*tu(profile(13),4) + tu(profile(13),1) )) && (u<=( time_sim_individual_cum(12) + 4*tu(profile(13),4) + tu(profile(13),2)))
             a_md =a_u_desired_backward(profile(13),2) ;
elseif (u>( time_sim_individual_cum (12)+ 4*tu(profile(13),4) + tu(profile(13),2) )) && (u<=( time_sim_individual_cum(12)+ 4*tu(profile(13),4) + tu(profile(13),3)))
             a_md =a_u_desired_backward(profile(13),3) ;   
elseif (u>( time_sim_individual_cum (12)+ 4*tu(profile(13),4) + tu(profile(13),3) )) && (u<=( time_sim_individual_cum(12)+ 4*tu(profile(13),4) + tu(profile(13),4)))
             a_md =a_u_desired_backward(profile(13),4) ;       
             
  
%% 14 14 14 14 14 14  %%%%%%%%%%%%%%       %%%%    %%%%              
             
elseif (u>(time_sim_individual_cum (13) + 0*tu(profile(14),4) + 0*tu(profile(12),1))) && (u<=(time_sim_individual_cum(13) + 0*tu(profile(14),4) + tu(profile(14),1)))
             a_md =a_u_desired_backward(profile(14),1) ;                  
elseif (u>( time_sim_individual_cum (13) + 0*tu(profile(14),4) + tu(profile(14),1) )) && (u<=( time_sim_individual_cum(13) + 0*tu(profile(14),4) + tu(profile(14),2)))
             a_md =a_u_desired_backward(profile(14),2) ;
elseif (u>( time_sim_individual_cum (13)+ 0*tu(profile(14),4) + tu(profile(14),2) )) && (u<=( time_sim_individual_cum(13)+ 0*tu(profile(14),4) + tu(profile(14),3)))
             a_md =a_u_desired_backward(profile(14),3) ;   
elseif (u>( time_sim_individual_cum (13)+ 0*tu(profile(14),4) + tu(profile(14),3) )) && (u<=( time_sim_individual_cum(13)+ 0*tu(profile(14),4) + tu(profile(14),4)))
             a_md =a_u_desired_backward(profile(14),4) ;    
             
elseif (u>(time_sim_individual_cum (13) + 1*tu(profile(14),4) + 0*tu(profile(12),1))) && (u<=(time_sim_individual_cum(13) + 1*tu(profile(14),4) + tu(profile(14),1)))
             a_md =a_u_desired_backward(profile(14),1) ;                  
elseif (u>( time_sim_individual_cum (13) + 1*tu(profile(14),4) + tu(profile(14),1) )) && (u<=( time_sim_individual_cum(13) + 1*tu(profile(14),4) + tu(profile(14),2)))
             a_md =a_u_desired_backward(profile(14),2) ;
elseif (u>( time_sim_individual_cum (13)+ 1*tu(profile(14),4) + tu(profile(14),2) )) && (u<=( time_sim_individual_cum(13)+ 1*tu(profile(14),4) + tu(profile(14),3)))
             a_md =a_u_desired_backward(profile(14),3) ;   
elseif (u>( time_sim_individual_cum (13)+ 1*tu(profile(14),4) + tu(profile(14),3) )) && (u<=( time_sim_individual_cum(13)+ 1*tu(profile(14),4) + tu(profile(14),4)))
             a_md =a_u_desired_backward(profile(14),4) ;      
             
elseif (u>(time_sim_individual_cum (13) + 2*tu(profile(14),4) + 0*tu(profile(12),1))) && (u<=(time_sim_individual_cum(13) + 2*tu(profile(14),4) + tu(profile(14),1)))
             a_md =a_u_desired_backward(profile(14),1) ;                  
elseif (u>( time_sim_individual_cum (13) + 2*tu(profile(14),4) + tu(profile(14),1) )) && (u<=( time_sim_individual_cum(13) + 2*tu(profile(14),4) + tu(profile(14),2)))
             a_md =a_u_desired_backward(profile(14),2) ;
elseif (u>( time_sim_individual_cum (13)+ 2*tu(profile(14),4) + tu(profile(14),2) )) && (u<=( time_sim_individual_cum(13)+ 2*tu(profile(14),4) + tu(profile(14),3)))
             a_md =a_u_desired_backward(profile(14),3) ;   
elseif (u>( time_sim_individual_cum (13)+ 2*tu(profile(14),4) + tu(profile(14),3) )) && (u<=( time_sim_individual_cum(13)+ 2*tu(profile(14),4) + tu(profile(14),4)))
             a_md =a_u_desired_backward(profile(14),4) ; 
             
elseif (u>(time_sim_individual_cum (13) + 3*tu(profile(14),4) + 0*tu(profile(12),1))) && (u<=(time_sim_individual_cum(13) + 3*tu(profile(14),4) + tu(profile(14),1)))
             a_md =a_u_desired_backward(profile(14),1) ;                  
elseif (u>( time_sim_individual_cum (13) + 3*tu(profile(14),4) + tu(profile(14),1) )) && (u<=( time_sim_individual_cum(13) + 3*tu(profile(14),4) + tu(profile(14),2)))
             a_md =a_u_desired_backward(profile(14),2) ;
elseif (u>( time_sim_individual_cum (13)+ 3*tu(profile(14),4) + tu(profile(14),2) )) && (u<=( time_sim_individual_cum(13)+ 3*tu(profile(14),4) + tu(profile(14),3)))
             a_md =a_u_desired_backward(profile(14),3) ;   
elseif (u>( time_sim_individual_cum (13)+ 3*tu(profile(14),4) + tu(profile(14),3) )) && (u<=( time_sim_individual_cum(13)+ 3*tu(profile(14),4) + tu(profile(14),4)))
             a_md =a_u_desired_backward(profile(14),4) ;   
             
elseif (u>(time_sim_individual_cum (13) + 4*tu(profile(14),4) + 0*tu(profile(12),1))) && (u<=(time_sim_individual_cum(13) + 4*tu(profile(14),4) + tu(profile(14),1)))
             a_md =a_u_desired_backward(profile(14),1) ;                  
elseif (u>( time_sim_individual_cum (13) + 4*tu(profile(14),4) + tu(profile(14),1) )) && (u<=( time_sim_individual_cum(13) + 4*tu(profile(14),4) + tu(profile(14),2)))
             a_md =a_u_desired_backward(profile(14),2) ;
elseif (u>( time_sim_individual_cum (13)+ 4*tu(profile(14),4) + tu(profile(14),2) )) && (u<=( time_sim_individual_cum(13)+ 4*tu(profile(14),4) + tu(profile(14),3)))
             a_md =a_u_desired_backward(profile(14),3) ;   
elseif (u>( time_sim_individual_cum (13)+ 4*tu(profile(14),4) + tu(profile(14),3) )) && (u<=( time_sim_individual_cum(13)+ 4*tu(profile(14),4) + tu(profile(14),4)))
             a_md =a_u_desired_backward(profile(14),4) ;              
             
             
             
%% 15 15 15 15 15 15  %%%%%%%%%%%%%%       %%%%    %%%%              
             
             
             
elseif (u>(time_sim_individual_cum (14) + 0*tu(profile(15),4) + 0*tu(profile(12),1))) && (u<=(time_sim_individual_cum(14) + 0*tu(profile(15),4) + tu(profile(15),1)))
             a_md =a_u_desired_backward(profile(15),1) ;                  
elseif (u>( time_sim_individual_cum (14) + 0*tu(profile(15),4) + tu(profile(15),1) )) && (u<=( time_sim_individual_cum(14) + 0*tu(profile(15),4) + tu(profile(15),2)))
             a_md =a_u_desired_backward(profile(15),2) ;
elseif (u>( time_sim_individual_cum (14)+ 0*tu(profile(15),4) + tu(profile(15),2) )) && (u<=( time_sim_individual_cum(14)+ 0*tu(profile(15),4) + tu(profile(15),3)))
             a_md =a_u_desired_backward(profile(15),3) ;   
elseif (u>( time_sim_individual_cum (14)+ 0*tu(profile(15),4) + tu(profile(15),3) )) && (u<=( time_sim_individual_cum(14)+ 0*tu(profile(15),4) + tu(profile(15),4)))
             a_md =a_u_desired_backward(profile(15),4) ;   
             
elseif (u>(time_sim_individual_cum (14) + 1*tu(profile(15),4) + 0*tu(profile(12),1))) && (u<=(time_sim_individual_cum(14) + 1*tu(profile(15),4) + tu(profile(15),1)))
             a_md =a_u_desired_backward(profile(15),1) ;                  
elseif (u>( time_sim_individual_cum (14) + 1*tu(profile(15),4) + tu(profile(15),1) )) && (u<=( time_sim_individual_cum(14) + 1*tu(profile(15),4) + tu(profile(15),2)))
             a_md =a_u_desired_backward(profile(15),2) ;
elseif (u>( time_sim_individual_cum (14)+ 1*tu(profile(15),4) + tu(profile(15),2) )) && (u<=( time_sim_individual_cum(14)+ 1*tu(profile(15),4) + tu(profile(15),3)))
             a_md =a_u_desired_backward(profile(15),3) ;   
elseif (u>( time_sim_individual_cum (14)+ 1*tu(profile(15),4) + tu(profile(15),3) )) && (u<=( time_sim_individual_cum(14)+ 1*tu(profile(15),4) + tu(profile(15),4)))
             a_md =a_u_desired_backward(profile(15),4) ;  
             
elseif (u>(time_sim_individual_cum (14) + 2*tu(profile(15),4) + 0*tu(profile(12),1))) && (u<=(time_sim_individual_cum(14) + 2*tu(profile(15),4) + tu(profile(15),1)))
             a_md =a_u_desired_backward(profile(15),1) ;                  
elseif (u>( time_sim_individual_cum (14) + 2*tu(profile(15),4) + tu(profile(15),1) )) && (u<=( time_sim_individual_cum(14) + 2*tu(profile(15),4) + tu(profile(15),2)))
             a_md =a_u_desired_backward(profile(15),2) ;
elseif (u>( time_sim_individual_cum (14)+ 2*tu(profile(15),4) + tu(profile(15),2) )) && (u<=( time_sim_individual_cum(14)+ 2*tu(profile(15),4) + tu(profile(15),3)))
             a_md =a_u_desired_backward(profile(15),3) ;   
elseif (u>( time_sim_individual_cum (14)+ 2*tu(profile(15),4) + tu(profile(15),3) )) && (u<=( time_sim_individual_cum(14)+ 2*tu(profile(15),4) + tu(profile(15),4)))
             a_md =a_u_desired_backward(profile(15),4) ;      
             
elseif (u>(time_sim_individual_cum (14) + 3*tu(profile(15),4) + 0*tu(profile(12),1))) && (u<=(time_sim_individual_cum(14) + 3*tu(profile(15),4) + tu(profile(15),1)))
             a_md =a_u_desired_backward(profile(15),1) ;                  
elseif (u>( time_sim_individual_cum (14) + 3*tu(profile(15),4) + tu(profile(15),1) )) && (u<=( time_sim_individual_cum(14) + 3*tu(profile(15),4) + tu(profile(15),2)))
             a_md =a_u_desired_backward(profile(15),2) ;
elseif (u>( time_sim_individual_cum (14)+ 3*tu(profile(15),4) + tu(profile(15),2) )) && (u<=( time_sim_individual_cum(14)+ 3*tu(profile(15),4) + tu(profile(15),3)))
             a_md =a_u_desired_backward(profile(15),3) ;   
elseif (u>( time_sim_individual_cum (14)+ 3*tu(profile(15),4) + tu(profile(15),3) )) && (u<=( time_sim_individual_cum(14)+ 3*tu(profile(15),4) + tu(profile(15),4)))
             a_md =a_u_desired_backward(profile(15),4) ;             

             

%% 16 16 16 16 16 16  %%%%%%%%%%%%%%       %%%%    %%%%              
             
             
             
elseif (u>(time_sim_individual_cum (15) + 0*tu(profile(16),4) + 0*tu(profile(12),1))) && (u<=(time_sim_individual_cum(15) + 0*tu(profile(16),4) + tu(profile(16),1)))
             a_md =a_u_desired_backward(profile(16),1) ;                  
elseif (u>( time_sim_individual_cum (15) + 0*tu(profile(16),4) + tu(profile(16),1) )) && (u<=( time_sim_individual_cum(15) + 0*tu(profile(16),4) + tu(profile(16),2)))
             a_md =a_u_desired_backward(profile(16),2) ;
elseif (u>( time_sim_individual_cum (15)+ 0*tu(profile(16),4) + tu(profile(16),2) )) && (u<=( time_sim_individual_cum(15)+ 0*tu(profile(16),4) + tu(profile(16),3)))
             a_md =a_u_desired_backward(profile(16),3) ;   
elseif (u>( time_sim_individual_cum (15)+ 0*tu(profile(16),4) + tu(profile(16),3) )) && (u<=( time_sim_individual_cum(15)+ 0*tu(profile(16),4) + tu(profile(16),4)))
             a_md =a_u_desired_backward(profile(16),4) ;
             
elseif (u>(time_sim_individual_cum (15) + 1*tu(profile(16),4) + 0*tu(profile(12),1))) && (u<=(time_sim_individual_cum(15) + 1*tu(profile(16),4) + tu(profile(16),1)))
             a_md =a_u_desired_backward(profile(16),1) ;                  
elseif (u>( time_sim_individual_cum (15) + 1*tu(profile(16),4) + tu(profile(16),1) )) && (u<=( time_sim_individual_cum(15) + 1*tu(profile(16),4) + tu(profile(16),2)))
             a_md =a_u_desired_backward(profile(16),2) ;
elseif (u>( time_sim_individual_cum (15)+ 1*tu(profile(16),4) + tu(profile(16),2) )) && (u<=( time_sim_individual_cum(15)+ 1*tu(profile(16),4) + tu(profile(16),3)))
             a_md =a_u_desired_backward(profile(16),3) ;   
elseif (u>( time_sim_individual_cum (15)+ 1*tu(profile(16),4) + tu(profile(16),3) )) && (u<=( time_sim_individual_cum(15)+ 1*tu(profile(16),4) + tu(profile(16),4)))
             a_md =a_u_desired_backward(profile(16),4) ;    
             
elseif (u>(time_sim_individual_cum (15) + 2*tu(profile(16),4) + 0*tu(profile(12),1))) && (u<=(time_sim_individual_cum(15) + 2*tu(profile(16),4) + tu(profile(16),1)))
             a_md =a_u_desired_backward(profile(16),1) ;                  
elseif (u>( time_sim_individual_cum (15) + 2*tu(profile(16),4) + tu(profile(16),1) )) && (u<=( time_sim_individual_cum(15) + 2*tu(profile(16),4) + tu(profile(16),2)))
             a_md =a_u_desired_backward(profile(16),2) ;
elseif (u>( time_sim_individual_cum (15)+ 2*tu(profile(16),4) + tu(profile(16),2) )) && (u<=( time_sim_individual_cum(15)+ 2*tu(profile(16),4) + tu(profile(16),3)))
             a_md =a_u_desired_backward(profile(16),3) ;   
elseif (u>( time_sim_individual_cum (15)+ 2*tu(profile(16),4) + tu(profile(16),3) )) && (u<=( time_sim_individual_cum(15)+ 2*tu(profile(16),4) + tu(profile(16),4)))
             a_md =a_u_desired_backward(profile(16),4) ;  
             
elseif (u>(time_sim_individual_cum (15) + 3*tu(profile(16),4) + 0*tu(profile(12),1))) && (u<=(time_sim_individual_cum(15) + 3*tu(profile(16),4) + tu(profile(16),1)))
             a_md =a_u_desired_backward(profile(16),1) ;                  
elseif (u>( time_sim_individual_cum (15) + 3*tu(profile(16),4) + tu(profile(16),1) )) && (u<=( time_sim_individual_cum(15) + 3*tu(profile(16),4) + tu(profile(16),2)))
             a_md =a_u_desired_backward(profile(16),2) ;
elseif (u>( time_sim_individual_cum (15)+ 3*tu(profile(16),4) + tu(profile(16),2) )) && (u<=( time_sim_individual_cum(15)+ 3*tu(profile(16),4) + tu(profile(16),3)))
             a_md =a_u_desired_backward(profile(16),3) ;   
elseif (u>( time_sim_individual_cum (15)+ 3*tu(profile(16),4) + tu(profile(16),3) )) && (u<=( time_sim_individual_cum(15)+ 3*tu(profile(16),4) + tu(profile(16),4)))
             a_md =a_u_desired_backward(profile(16),4) ;   
             
elseif (u>(time_sim_individual_cum (15) + 4*tu(profile(16),4) + 0*tu(profile(12),1))) && (u<=(time_sim_individual_cum(15) + 4*tu(profile(16),4) + tu(profile(16),1)))
             a_md =a_u_desired_backward(profile(16),1) ;                  
elseif (u>( time_sim_individual_cum (15) + 4*tu(profile(16),4) + tu(profile(16),1) )) && (u<=( time_sim_individual_cum(15) + 4*tu(profile(16),4) + tu(profile(16),2)))
             a_md =a_u_desired_backward(profile(16),2) ;
elseif (u>( time_sim_individual_cum (15)+ 4*tu(profile(16),4) + tu(profile(16),2) )) && (u<=( time_sim_individual_cum(15)+ 4*tu(profile(16),4) + tu(profile(16),3)))
             a_md =a_u_desired_backward(profile(16),3) ;   
elseif (u>( time_sim_individual_cum (15)+ 4*tu(profile(16),4) + tu(profile(16),3) )) && (u<=( time_sim_individual_cum(15)+ 4*tu(profile(16),4) + tu(profile(16),4)))
             a_md =a_u_desired_backward(profile(16),4) ;  
             
elseif (u>(time_sim_individual_cum (15) + 5*tu(profile(16),4) + 0*tu(profile(12),1))) && (u<=(time_sim_individual_cum(15) + 5*tu(profile(16),4) + tu(profile(16),1)))
             a_md =a_u_desired_backward(profile(16),1) ;                  
elseif (u>( time_sim_individual_cum (15) + 5*tu(profile(16),4) + tu(profile(16),1) )) && (u<=( time_sim_individual_cum(15) + 5*tu(profile(16),4) + tu(profile(16),2)))
             a_md =a_u_desired_backward(profile(16),2) ;
elseif (u>( time_sim_individual_cum (15)+ 5*tu(profile(16),4) + tu(profile(16),2) )) && (u<=( time_sim_individual_cum(15)+ 5*tu(profile(16),4) + tu(profile(16),3)))
             a_md =a_u_desired_backward(profile(16),3) ;   
elseif (u>( time_sim_individual_cum (15)+ 5*tu(profile(16),4) + tu(profile(16),3) )) && (u<=( time_sim_individual_cum(15)+ 5*tu(profile(16),4) + tu(profile(16),4)))
             a_md =a_u_desired_backward(profile(16),4) ;                
             
else
        a_md = a_u_desired(profile(1),4) ;
end
